simulink model "flyback_switching_average_2017a"  (R2017a)
settings: Solver=ode23tb  StartTime=0.0  StopTime=.02  RelTol=1e-4
values from neighbouring files (symbols this model uses):
  D = (V)/(Vg-(Iout*Rg))    (= 0.447204968944)    [lsm.m]
  Ts = 1/fsw    (= 1e-05)    [lsm.m]
  V = 12    [lsm.m]
  Vg = 28    [lsm.m]
undefined symbols (not defined in the file or in its folder): Cout, Imag, Lm, n, Ron, Rout
libraries: powerlib x19
settings Model: Creator=jvr2131  LastModifiedBy=jvr2131
settings DataIOCC: LimitDataPoints=on  SaveFormat=Array
settings OptimizationCC: BlockReduction=off  BooleanDataType=off  LifeSpan=inf
settings DebuggingCC: SaveWithParameterizedLinksMsg=none  UnderspecifiedInitializationDetection=Classic  MergeDetectMultiDrivingBlocksExec=none  SignalResolutionControl=TryResolveAllWithWarning  MultiTaskDSMMsg=warning  MultiTaskCondExecSysMsg=none  StateNameClashWarn=warning  StrictBusMsg=None  SFUnexpectedBacktrackingDiag=warning  SFNoUnconditionalDefaultTransitionDiag=warning  SFExecutionAtInitializationDiag=none
settings HardwareCC: ProdBitPerPointer=32  ProdBitPerSizeT=32  ProdBitPerPtrDiffT=32  ProdLargestAtomicFloat=None  ProdIntDivRoundTo=Undefined  ProdEndianess=Unspecified  ProdWordSize=32  ProdHWDeviceType=32-bit Generic  TargetUnknown=on
settings ModelReferenceCC: PropagateSignalLabelsOutOfModel=off
settings GRTTargetCC: TargetLangStandard=C89/C90 (ANSI)  GeneratePreprocessorConditionals=Disable all
settings ConfigComp: CovMetricSettings=dw  CovHtmlReporting=on  CovSaveCumulativeToWorkspaceVar=on  CovSaveSingleToWorkspaceVar=on  CovExternalEMLEnable=off
settings SimscapeCC: SimscapeNormalizeSystem=off

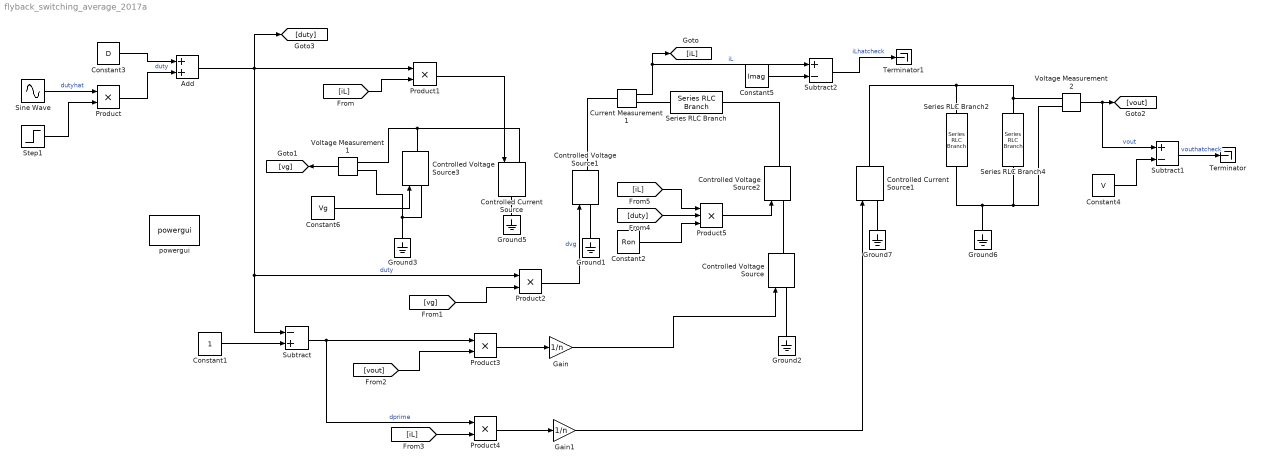
== system flyback_switching_average_2017a ==
  Add : Sum
  Constant1 : Constant
  Constant2 : Constant  Value=Ron
  Constant3 : Constant  Value=D
  Constant4 : Constant  Value=V
  Constant5 : Constant  Value=Imag
  Constant6 : Constant  Value=Vg
  Controlled Current Source : powerlib/Electrical Sources/Controlled Current Source  Initialize=on  Source_Type=AC  Amplitude=0  Phase=0  Frequency=0  Measurements=None
  Controlled Current Source1 : powerlib/Electrical Sources/Controlled Current Source  Initialize=on  Source_Type=AC  Amplitude=0  Phase=0  Frequency=0  Measurements=None
  Controlled Voltage Source{,1..3} (4 alike) : powerlib/Electrical Sources/Controlled Voltage Source  Initialize=on  Source_Type=AC  Amplitude=0  Phase=0  Frequency=0  Measurements=None
  Current Measurement1 : powerlib/Measurements/Current Measurement  PhasorSimulation=off  OutputType=Complex  PSBequivalent=0
  Gain : Gain  Gain=1/n
  Gain1 : Gain  Gain=1/n
  Ground{1..3,5..7} (6 alike) : powerlib/Elements/Ground  LConnTagsString=a
  Product{,1..4} (5 alike) : Product
  Product5 : Product  Inputs=3
  Series RLC Branch : powerlib/Elements/Series RLC Branch  LConnTagsString=__new0  RConnTagsString=__new0  BranchType=L  Resistance=1  Inductance=Lm  SetiL0=off  InitialCurrent=0  Capacitance=1e-6  Setx0=off  InitialVoltage=0  Measurements=None
  Series RLC Branch2 : powerlib/Elements/Series RLC Branch  LConnTagsString=__new0  RConnTagsString=__new0  BranchType=C  Resistance=1  Inductance=1e-3  SetiL0=off  InitialCurrent=0  Capacitance=Cout  Setx0=off  InitialVoltage=0  Measurements=None
  Series RLC Branch4 : powerlib/Elements/Series RLC Branch  LConnTagsString=__new0  RConnTagsString=__new0  BranchType=R  Resistance=Rout  Inductance=1e-3  SetiL0=off  InitialCurrent=0  Capacitance=Cout  Setx0=off  InitialVoltage=0  Measurements=None
  Sine Wave : Sin  Amplitude=.01  Frequency=2*pi*1000  SampleTime=0
  Step1 : Step  Time=10e-3  SampleTime=0
  Subtract : Sum  Inputs=-+
  Subtract1 : Sum  Inputs=+-
  Subtract2 : Sum  Inputs=+-
  Terminator : Terminator
  Terminator1 : Terminator
  Voltage Measurement1 : powerlib/Measurements/Voltage Measurement  PhasorSimulation=off  OutputType=Complex  PSBequivalent=0
  Voltage Measurement2 : powerlib/Measurements/Voltage Measurement  PhasorSimulation=off  OutputType=Complex  PSBequivalent=0
  powergui : powerlib/powergui  Priority=1  SimulationMode=Continuous  SampleTime=Ts/1000  frequency=60  Iterations=50  frequencyindice=0  Pbase=100e6  ErrMax=1e-4  UnitsV=kV  UnitsW=MW  buscounter=0  FunctionMessages=off  echomessages=off  EnableUseOfTLC=off  CurrentSourceSwitches=off  DisableSnubberDevices=off  DisableRonSwitches=off  DisableVfSwitches=off  DisplayEquations=off  SolverType=Tustin  Interpol=off  ExternalGateDelay=off  methode=off  Ts=0  x0status=blocks  SPID=off  SwTol=0  HookPort=off  RestoreLinks=warning  ResistiveCurrentMeasurement=off  Frange=[0:2:500]  Ylog=off  Xlog=on  ShowGrid=off  save=off  variable=ZData  structure=0  ZoomFFT=off  StartTime=0.0  cycles=1  DisplayStyle=1  fundamental=60  FreqAxis=off  MaxFrequency=1000  frequencyindicesteady=1  RmsSteady=1  display=off
  wires:
  Add/1 -> [duty], Subtract/1, Product2/1, Product1/1  "duty"
  Current Measurement1/1 -> Subtract2/1, [iL]  "iL"
  Voltage Measurement1/1 -> [vg]
  Voltage Measurement2/1 -> Subtract1/1, [vout]  "vout"
  [iL] -> Product1/2
  Product1/1 -> Controlled Current Source/1
  [vg] -> Product2/2
  Product2/1 -> Controlled Voltage Source1/1  "dvg"
  Constant1/1 -> Subtract/2
  Subtract/1 -> Product4/1, Product3/1  "dprime"
  [vout] -> Product3/2
  Product3/1 -> Gain/1
  Gain/1 -> Controlled Voltage Source/1
  [iL] -> Product4/2
  Product4/1 -> Gain1/1
  Gain1/1 -> Controlled Current Source1/1
  [duty] -> Product5/2
  [iL] -> Product5/1
  Constant2/1 -> Product5/3
  Product5/1 -> Controlled Voltage Source2/1
  Step1/1 -> Product/2
  Sine Wave/1 -> Product/1  "dutyhat"
  Product/1 -> Add/2  "duty"
  Constant3/1 -> Add/1
  Constant4/1 -> Subtract1/2
  Subtract1/1 -> Terminator/1  "vouthatcheck"
  Constant5/1 -> Subtract2/2
  Subtract2/1 -> Terminator1/1  "iLhatcheck"
  Constant6/1 -> Controlled Voltage Source3/1
  connections:
  Ground1/LConn1 -- Controlled Voltage Source1/LConn1
  Ground2/LConn1 -- Controlled Voltage Source/LConn1
  Voltage Measurement1/LConn1 -- Controlled Voltage Source3/RConn1 -- Controlled Current Source/LConn1
  Voltage Measurement1/LConn2 -- Controlled Voltage Source3/LConn1 -- Ground3/LConn1
  Ground5/LConn1 -- Controlled Current Source/RConn1
  Current Measurement1/RConn1 -- Series RLC Branch/LConn1
  Current Measurement1/LConn1 -- Controlled Voltage Source1/RConn1
  Series RLC Branch4/LConn1 -- Voltage Measurement2/LConn2 -- Ground6/LConn1 -- Series RLC Branch2/RConn1
  Series RLC Branch2/LConn1 -- Voltage Measurement2/LConn1 -- Series RLC Branch4/RConn1 -- Controlled Current Source1/RConn1
  Ground7/LConn1 -- Controlled Current Source1/LConn1
  Controlled Voltage Source2/LConn1 -- Controlled Voltage Source/RConn1
  Controlled Voltage Source2/RConn1 -- Series RLC Branch/RConn1
